simulink library "Lib_Turbo_TurbinePSI_TMATS"  (R2012b)
settings: Solver=ode45  StartTime=0.0  StopTime=10.0  RelTol=1e-3
libraries: Lib_Solve_DataOut_TMATS x4
Description:
  | Thomas Modules
settings Model: Creator=jwchapm2  LastModifiedBy=jwchapm2

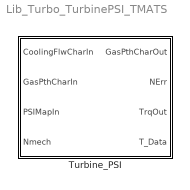
== system Lib_Turbo_TurbinePSI_TMATS ==
  Turbine_PSI : Subsystem  mask(T-MATS: Turbine_PSI Library Block){X_T_PRpVec_M=[ 3.000  8.000], Y_T_NcpVec_M=[60 80  110], T_T_Map_PSIArray_M=[0 0; 0 0; 0 0], X_T_PRwVec_M=[60 80  110], Y_T_NcwVec_M=[60 80  110], T_T_Map_WoWArray_M=[0 0;0 0; 0 0], s_T_hi_M=0.1, s_T_Nc_M=0.0243, s_T_Wc_M=0.4504, s_T_PR_M=0.9736, s_T_Eff_M=0.9984, CFlwEn_M=off, T_CoolFlwPos_M=0, gamma_M=1.4, Rt_M=0.1, iDesign_M=2, NcDes_M=100, EffDes_M=0.9328, PRDes_M=5, NDes_M=10000, FVar_M='iDesScalars.mat', SVar_M=gcb, NcNm_M='_C_Nc', WcNm_M='_C_Wc', PRNm_M='_C_PR', EffNm_M='_C_Eff'}
      mask prompts: X_T_PRpVec_M "X_T_PRpVec_M - Turbine Map Pressure Ratio Vector (X-axis)(nx1)"; Y_T_NcpVec_M "Y_T_NcpVec_M - Turbine Map Corrected Speed Vector (Y-axis)(mx1)"; T_T_Map_PSIArray_M "T_T_Map_PSIArray_M - Turbine Map PSIMAPI Array (PSIMAPI = f(Nc,PR))(mxn)"; X_T_PRwVec_M "X_T_PRwVec_M - Turbine Map Pressure Ratio Vector (X-axis)(rx1)"; Y_T_NcwVec_M "Y_T_NcwVec_M - Turbine Map Corrected Speed Vector (Y-axis)(qx1)"; T_T_Map_WoWArray_M "T_T_Map_WoWArray_M - Turbine Map Flow Array (WoW=f(Nc,PR))(qxr)"; s_T_hi_M "s_T_hi_M - Corrected Entalpy Constant (T_hi)"; s_T_Nc_M "s_T_Nc_M - Corrected Speed Scalar Constant (T_Nc)"; s_T_Wc_M "s_T_Wc_M - Flow Scalar Constant (T_Wc)"; s_T_PR_M "s_T_PR_M - Pressure Ratio Scalar Constant (T_PR)"; s_T_Eff_M "s_T_Eff_M - Efficiency Scalar Constant (T_Eff)"; CFlwEn_M "CFlwEn_M - Cooling Flow Enable [0-off, 1-on]"; T_CoolFlwPos_M "T_CoolFlwPos_M - Cooling Flow position [0 at inlet,  1 at exit] (cx1)"; iDesign_M "iDesign_M - Design fork (0 - Enable iDes, 1 - Use iDes Scalars, 2 - Use Specified Input Scalars)"; NcDes_M "NcDes_M - Design Corrected Shaft Speed [rpm]"; EffDes_M "EffDes_M - Design Efficiency [frac]"; PRDes_M "PRDes_M - Design Pressure Ratio [frac]"; NDes_M "NDes_M - Design Shaft Speed [rpm]"; FVar_M "FVar_M - File name for iDes Variables"; SVar_M "SVar_M - iDes Variable Surname"; NcNm_M "NcNm_M - iDes Nc scalar variable name"; WcNm_M "WcNm_M - iDes Wc scalar variable name"; PRNm_M "PRNm_M - iDes PR scalar variable name"; EffNm_M "EffNm_M - iDes Eff scalar variable name"
      mask help: This block simulates the performance of a turbine using basic thermodynamic equations, properties, and table lookups. Turbine_PSI look up tables for this block are based on PSI instead Pressure Ratio as in the Turbine block.
      mask init:
      | if iDesign_M == 1
      |     load(FVar_M);
      |     s_T_Nc_M = eval(strcat(stripchar_TMATS(SVar_M),NcNm_M));
      |     s_T_Wc_M = eval(strcat(stripchar_TMATS(SVar_M),WcNm_M));
      |     s_T_PR_M = eval(strcat(stripchar_TMATS(SVar_M),PRNm_M));
      |     s_T_Eff_M = eval(strcat(stripchar_TMATS(SVar_M),EffNm_M));
      | end
      mask Help: web(which('Turbo_TMATS_TrbPSI.html'),'-helpbrowser')
      mask Callback CFlwEn_M: MSK_SEC_Enables_TMATS('CFlwEn_M',13,'en')
      mask Callback iDesign_M:
      | MSK_SEC_Enables_Ides_TMATS('iDesign_M',[8 9 10 11],'G1')
      | MSK_SEC_Enables_Ides_TMATS('iDesign_M',[17 18 19 20],'G2')
      | MSK_SEC_Enables_Ides_TMATS('iDesign_M',[21 22 23 24 25 26],'G3')

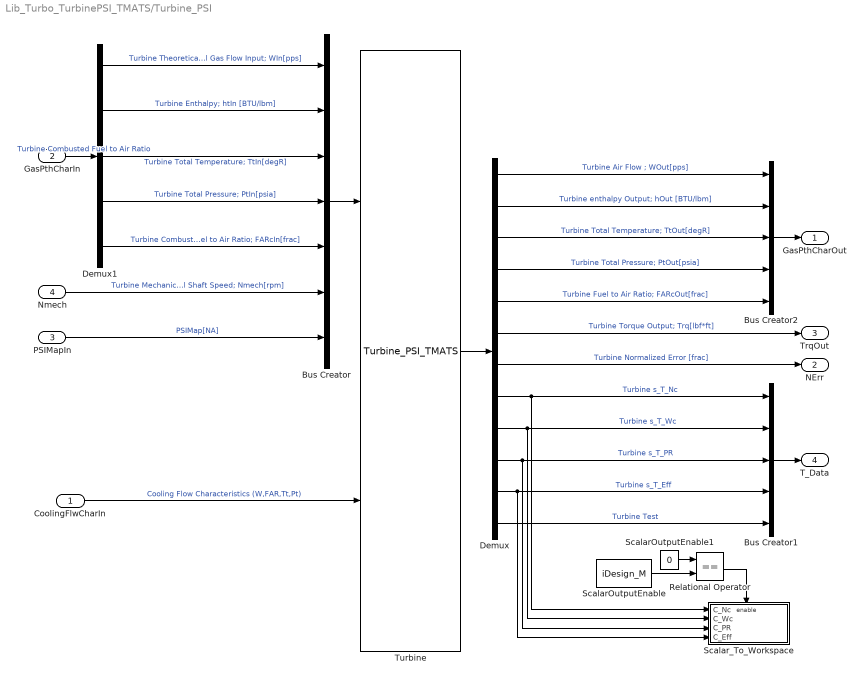
== system Lib_Turbo_TurbinePSI_TMATS/Turbine_PSI ==
  CoolingFlwCharIn : Inport
  GasPthCharIn : Inport  Port=2
  PSIMapIn : Inport  Port=3
  Nmech : Inport  Port=4
  Bus Creator : BusCreator  Inputs=7
  Bus Creator1 : BusCreator  Inputs=5
  Bus Creator2 : BusCreator  Inputs=5
  Demux : Demux  Outputs=12
  Demux1 : Demux  Outputs=5
  Relational Operator : RelationalOperator  Operator===  OutDataTypeStr=boolean
  ScalarOutputEnable : Constant  Value=iDesign_M
  ScalarOutputEnable1 : Constant  Value=0
  Scalar_To_Workspace : Subsystem
  Turbine : S-Function  FunctionName=Turbine_PSI_TMATS  Parameters=s_T_Nc_M, s_T_PR_M, s_T_Wc_M, s_T_Eff_M, Y_T_NcpVec_M, X_T_PRpVec_M, Y_T_NcwVec_M, X_T_PRwVec_M, T_T_Map_WoWArray_M, T_T_Map_PSIArray_M, T_CoolFlwPos_M, length(T_CoolFlwPos_M), CFlwEn_M, iDesign_M, NcDes_M, EffDes_M, PRDes_M, NDes_M, s_T_hi_M, gamma_M, Rt_M, gcs  EnableBusSupport=off
  GasPthCharOut : Outport
  NErr : Outport  Port=2
  TrqOut : Outport  Port=3
  T_Data : Outport  Port=4
  wires:
  Demux/11 -> Scalar_To_Workspace/4(C_Eff), Bus Creator1/4  "Turbine s_T_Eff"
  Demux/10 -> Scalar_To_Workspace/3(C_PR), Bus Creator1/3  "Turbine s_T_PR"
  Demux/9 -> Scalar_To_Workspace/2(C_Wc), Bus Creator1/2  "Turbine s_T_Wc"
  Demux/8 -> Scalar_To_Workspace/1(C_Nc), Bus Creator1/1  "Turbine s_T_Nc"
  Bus Creator1/1 -> T_Data/1
  Demux1/5 -> Bus Creator/5  "Turbine Combusted Fuel to Air Ratio; FARcIn[frac]"
  CoolingFlwCharIn/1 -> Turbine/2  "Cooling Flow Characteristics (W,FAR,Tt,Pt)"
  Demux/7 -> NErr/1  "Turbine Normalized Error [frac]"
  Demux1/1 -> Bus Creator/1  "Turbine Theoretical Gas Flow Input; WIn[pps]"
  GasPthCharIn/1 -> Demux1/1  "Turbine Combusted Fuel to Air Ratio"
  Bus Creator2/1 -> GasPthCharOut/1
  Demux1/4 -> Bus Creator/4  "Turbine Total Pressure; PtIn[psia]"
  Nmech/1 -> Bus Creator/6  "Turbine Mechanical Shaft Speed; Nmech[rpm]"
  Demux/6 -> TrqOut/1  "Turbine Torque Output; Trq[lbf*ft]"
  Demux/2 -> Bus Creator2/2  "Turbine enthalpy Output; hOut [BTU/lbm]"
  Bus Creator/1 -> Turbine/1
  Demux/4 -> Bus Creator2/4  "Turbine Total Pressure; PtOut[psia]"
  Demux/3 -> Bus Creator2/3  "Turbine Total Temperature; TtOut[degR]"
  Demux/5 -> Bus Creator2/5  "Turbine Fuel to Air Ratio; FARcOut[frac]"
  Demux/1 -> Bus Creator2/1  "Turbine Air Flow ; WOut[pps]"
  Turbine/1 -> Demux/1
  Demux1/3 -> Bus Creator/3  "Turbine Total Temperature; TtIn[degR]"
  Demux1/2 -> Bus Creator/2  "Turbine Enthalpy; htIn [BTU/lbm]"
  PSIMapIn/1 -> Bus Creator/7  "PSIMap[NA]"
  Demux/12 -> Bus Creator1/5  "Turbine Test"
  ScalarOutputEnable/1 -> Relational Operator/2
  ScalarOutputEnable1/1 -> Relational Operator/1
  Relational Operator/1 -> Scalar_To_Workspace/Enable

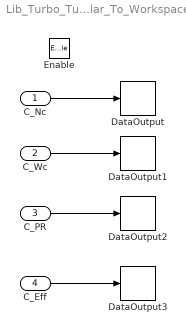
== system Lib_Turbo_TurbinePSI_TMATS/Turbine_PSI/Scalar_To_Workspace ==
  C_Nc : Inport
  C_Wc : Inport  Port=2
  C_PR : Inport  Port=3
  C_Eff : Inport  Port=4
  Enable : EnablePort
  DataOutput : Lib_Solve_DataOut_TMATS/DataOutput  FVar_M=FVar_M  Var_M=NcNm_M  SVar_M=SVar_M
  DataOutput1 : Lib_Solve_DataOut_TMATS/DataOutput  FVar_M=FVar_M  Var_M=WcNm_M  SVar_M=SVar_M
  DataOutput2 : Lib_Solve_DataOut_TMATS/DataOutput  FVar_M=FVar_M  Var_M=PRNm_M  SVar_M=SVar_M
  DataOutput3 : Lib_Solve_DataOut_TMATS/DataOutput  FVar_M=FVar_M  Var_M=EffNm_M  SVar_M=SVar_M
  wires:
  C_Eff/1 -> DataOutput3/1
  C_PR/1 -> DataOutput2/1
  C_Wc/1 -> DataOutput1/1
  C_Nc/1 -> DataOutput/1
